simulink model "washout5useful"  (R2018b)
settings: Solver=VariableStepAuto  StartTime=0.0  StopTime=20  RelTol=1e-3
undefined symbols (not defined in the file or in its folder): sigbuilder_block
libraries: fuzblock x2
settings Model: Creator=15705  LastModifiedBy=15705

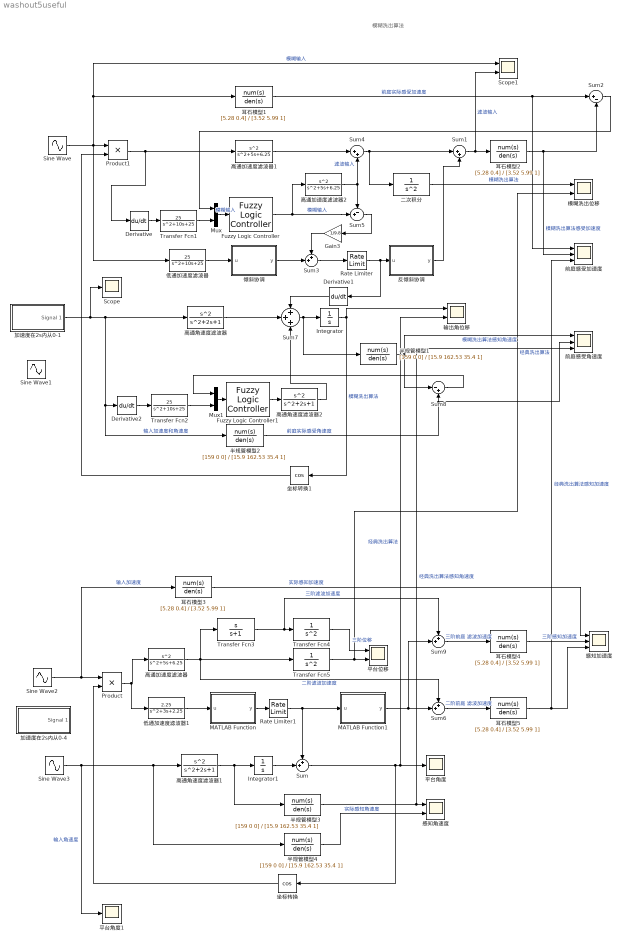
== system washout5useful ==
  note: 模糊洗出算法
  Derivative : Derivative
  Derivative1 : Derivative
  Derivative2 : Derivative
  Fuzzy Logic Controller : fuzblock/Fuzzy Logic  Controller  FIS=InputFuzzy  OutputSampleNumber=101  DataType=double  FuzzifiedInputs=off  RuleFiringStrengths=off  RuleOutputs=off  AggregatedOutputs=off  SimulateUsing=Interpreted execution  OutOfRangeInputValueMessage=warning  NoRuleFiredMessage=warning  EmptyOutputFuzzySetMessage=warning
  Fuzzy Logic Controller1 : fuzblock/Fuzzy Logic  Controller  FIS=Input_ang  OutputSampleNumber=101  DataType=double  FuzzifiedInputs=off  RuleFiringStrengths=off  RuleOutputs=off  AggregatedOutputs=off  SimulateUsing=Interpreted execution  OutOfRangeInputValueMessage=warning  NoRuleFiredMessage=warning  EmptyOutputFuzzySetMessage=warning
  Gain3 : Gain  Gain=1/9.8
  Integrator : Integrator
  Integrator1 : Integrator
  MATLAB Function : MATLAB Function  TreatAsAtomicUnit=on
  MATLAB Function1 : MATLAB Function  TreatAsAtomicUnit=on
  Mux : Mux  Inputs=2
  Mux1 : Mux  Inputs=2
  Product : Product
  Product1 : Product
  Rate Limiter : RateLimiter  RisingSlewLimit=0.0628  FallingSlewLimit=-0.0628  SampleTimeMode=inherited
  Rate Limiter1 : RateLimiter  RisingSlewLimit=0.0628  FallingSlewLimit=-0.0628  SampleTimeMode=inherited
  Scope : Scope
  Scope1 : Scope  NumInputPorts=2
  Sine Wave{,1..3} (4 alike) : Sin  SampleTime=0
  Sum{,3,6,9} (4 alike) : Sum  Inputs=++|
  Sum1 : Sum  Inputs=|++
  Sum2 : Sum  Inputs=|+-
  Sum4 : Sum  Inputs=|++
  Sum5 : Sum  Inputs=-+|
  Sum7 : Sum  Inputs=+++
  Sum8 : Sum  Inputs=|-+
  Transfer Fcn1 : TransferFcn  Numerator=[25]  Denominator=[1 10 25]
  Transfer Fcn2 : TransferFcn  Numerator=[25]  Denominator=[1 10 25]
  Transfer Fcn3 : TransferFcn  Numerator=[1 0]  Denominator=[1 1]
  Transfer Fcn4 : TransferFcn  Denominator=[1 0 0]
  Transfer Fcn5 : TransferFcn  Denominator=[1 0 0]
  二次积分 : TransferFcn  Denominator=[1 0 0]
  低通加速度滤波器 : TransferFcn  Numerator=[25]  Denominator=[1 10 25]
  低通加速度滤波器1 : TransferFcn  Numerator=[2.25]  Denominator=[1 3 2.25]
  倾斜协调 : MATLAB Function  TreatAsAtomicUnit=on
  前庭感受加速度 : Scope  NumInputPorts=3
  前庭感受角速度 : Scope  NumInputPorts=3
  加速度在2s内从0-1 : Subsystem  Tag=STV Subsys  LoadFcn=sigbuilder_block('load');  StartFcn=sigbuilder_block('start');  StopFcn=sigbuilder_block('stop');  ClipboardFcn=sigbuilder_block('clipboard');  mask(Sigbuilder block){tuvar=[0:10]}
      mask help: Simulink:masks:SigbuilderBlock_MD
      mask init:
      | if ~strcmp(get_param(bdroot(gcbh),'SimulationStatus'),'stopped') tuvar = sigbuilder_block('maskInit'); end
      settings: CopyFcn=sigbuilder_block('copy');  DeleteFcn=sigbuilder_block('delete');  ModelCloseFcn=sigbuilder_block('modelClose');  PreSaveFcn=sigbuilder_block('preSave');  PauseFcn=sigbuilder_block('pause');  ContinueFcn=sigbuilder_block('continue');  NameChangeFcn=sigbuilder_block('namechange');  OpenFcn=sigbuilder_block('open',[199.875 127.5 550.5 364.5 ]);  CloseFcn=sigbuilder_block('close');
      mask Display: plot(0, 0, 100, 100,[2, 2, 32, 32, 2], [68, 8, 8, 68, 68],[32, 2], [38, 38], [32, 19, 2],[53, 60, 44], [32, 17, 17, 2],[16, 16, 31, 31]);txt = getActiveGroup(gcbh);text(2, 100, txt,'verticalAlignment', 'top');
  加速度在2s内从0-4 : Subsystem  Tag=STV Subsys  LoadFcn=sigbuilder_block('load');  StartFcn=sigbuilder_block('start');  StopFcn=sigbuilder_block('stop');  ClipboardFcn=sigbuilder_block('clipboard');  mask(Sigbuilder block){tuvar=[0:10]}
      mask help: Simulink:masks:SigbuilderBlock_MD
      mask init:
      | if ~strcmp(get_param(bdroot(gcbh),'SimulationStatus'),'stopped') tuvar = sigbuilder_block('maskInit'); end
      settings: CopyFcn=sigbuilder_block('copy');  DeleteFcn=sigbuilder_block('delete');  ModelCloseFcn=sigbuilder_block('modelClose');  PreSaveFcn=sigbuilder_block('preSave');  PauseFcn=sigbuilder_block('pause');  ContinueFcn=sigbuilder_block('continue');  NameChangeFcn=sigbuilder_block('namechange');  OpenFcn=sigbuilder_block('open',[199.875 127.5 550.5 364.5 ]);  CloseFcn=sigbuilder_block('close');
      mask Display: plot(0, 0, 100, 100,[2, 2, 32, 32, 2], [68, 8, 8, 68, 68],[32, 2], [38, 38], [32, 19, 2],[53, 60, 44], [32, 17, 17, 2],[16, 16, 31, 31]);txt = getActiveGroup(gcbh);text(2, 100, txt,'verticalAlignment', 'top');
  半规管模型{1..4} (4 alike) : TransferFcn  Numerator=[159 0 0]  Denominator=[15.9 162.53 35.4 1]
  反倾斜协调 : MATLAB Function  TreatAsAtomicUnit=on
  坐标转换 : Trigonometry  Operator=cos
  坐标转换1 : Trigonometry  Operator=cos
  平台位移 : Scope  NumInputPorts=2
  平台角度 : Scope
  平台角度1 : Scope
  感知加速度 : Scope  NumInputPorts=3
  感知角速度 : Scope  NumInputPorts=2
  模糊洗出位移 : Scope  NumInputPorts=2
  耳石模型{1..5} (5 alike) : TransferFcn  Numerator=[5.28 0.4]  Denominator=[3.52 5.99 1]
  "输出角位移 " : Scope  NumInputPorts=2
  高通加速度滤波器 : TransferFcn  Numerator=[1 0 0]  Denominator=[1 5 6.25]
  高通加速度滤波器1 : TransferFcn  Numerator=[1 0 0]  Denominator=[1 5 6.25]
  高通加速度滤波器2 : TransferFcn  Numerator=[1 0 0]  Denominator=[1 5 6.25]
  高通角速度滤波器 : TransferFcn  Numerator=[1 0 0]
  高通角速度滤波器1 : TransferFcn  Numerator=[1 0 0]
  高通角速度滤波器2 : TransferFcn  Numerator=[1 0 0]
  wires:
  Rate Limiter/1 -> Derivative1/1, 反倾斜协调/1(u)
  耳石模型2/1 -> Sum2/2, 前庭感受加速度/2  "模糊洗出算法感受加速度"
  二次积分/1 -> 模糊洗出位移/1  "模糊洗出算法"
  耳石模型1/1 -> Sum2/1, 前庭感受加速度/1  "前庭实际感受加速度"
  加速度在2s内从0-1/1(Signal 1) -> Scope/1, 高通角速度滤波器/1, Derivative2/1, 半规管模型2/1  "输入加速度和角速度"
  Sine Wave/1 -> Product1/1, 耳石模型1/1, Scope1/1, 低通加速度滤波器/1  "模糊输入"
  Integrator/1 -> 坐标转换1/1, "输出角位移 "/1  "模糊洗出算法"
  低通加速度滤波器/1 -> 倾斜协调/1(u)
  Mux/1 -> Fuzzy Logic Controller/1  "模糊输入"
  Fuzzy Logic Controller/1 -> 高通加速度滤波器2/1, Sum5/2  "模糊输入"
  倾斜协调/1(y) -> Sum3/2
  Sum3/1 -> Rate Limiter/1
  Derivative/1 -> Transfer Fcn1/1
  高通加速度滤波器1/1 -> Sum4/1
  Sum4/1 -> Sum1/1, 二次积分/1
  高通加速度滤波器2/1 -> Sum5/1, Sum4/2  "滤波输入"
  Sum5/1 -> Gain3/1
  反倾斜协调/1(y) -> Sum1/2
  Sum1/1 -> 耳石模型2/1, Scope1/2  "滤波输入"
  Gain3/1 -> Sum3/1
  Sum2/1 -> Mux/1
  Transfer Fcn1/1 -> Mux/2
  Sum7/1 -> Integrator/1, 半规管模型1/1
  高通角速度滤波器/1 -> Sum7/2
  Derivative1/1 -> Sum7/1
  半规管模型1/1 -> Sum8/1, 前庭感受角速度/1  "模糊洗出算法感知角速度"
  半规管模型2/1 -> 前庭感受角速度/2, Sum8/2  "前庭实际感受角速度"
  Mux1/1 -> Fuzzy Logic Controller1/1
  Derivative2/1 -> Transfer Fcn2/1
  Sum8/1 -> Mux1/1
  Fuzzy Logic Controller1/1 -> 高通角速度滤波器2/1
  高通角速度滤波器2/1 -> Sum7/3
  Transfer Fcn2/1 -> Mux1/2
  半规管模型4/1 -> 感知角速度/2  "实际感知角速度"
  MATLAB Function/1(y) -> Rate Limiter1/1
  高通角速度滤波器1/1 -> 半规管模型3/1, Integrator1/1
  Sum6/1 -> 耳石模型5/1  "二阶前庭 滤波加速度"
  耳石模型4/1 -> 感知加速度/2  "三阶感知加速度"
  低通加速度滤波器1/1 -> MATLAB Function/1(u)
  坐标转换/1 -> Product/2
  半规管模型3/1 -> 前庭感受角速度/3, 感知角速度/1  "经典洗出算法感知角速度"
  MATLAB Function1/1(y) -> Sum9/2, Sum6/2
  Sine Wave2/1 -> Product/1, 耳石模型3/1  "输入加速度"
  耳石模型5/1 -> 前庭感受加速度/3, 感知加速度/3  "经典洗出算法感知加速度"
  Transfer Fcn5/1 -> 模糊洗出位移/2, 平台位移/2  "经典洗出算法"
  耳石模型3/1 -> 感知加速度/1  "实际感知加速度"
  Sum9/1 -> 耳石模型4/1  "三阶前庭 滤波加速度"
  Transfer Fcn3/1 -> Sum9/1, Transfer Fcn4/1  "三阶滤波加速度"
  Integrator1/1 -> Sum/2
  Sine Wave3/1 -> 平台角度1/1, 半规管模型4/1, 高通角速度滤波器1/1  "输入角速度"
  Rate Limiter1/1 -> MATLAB Function1/1(u), Sum/1
  高通加速度滤波器/1 -> Transfer Fcn3/1, Sum6/1, Transfer Fcn5/1  "二阶滤波加速度"
  Product/1 -> 低通加速度滤波器1/1, 高通加速度滤波器/1
  Transfer Fcn4/1 -> 平台位移/1  "三阶位移"
  Sum/1 -> "输出角位移 "/2, 平台角度/1, 坐标转换/1  "经典洗出算法"
  坐标转换1/1 -> Product1/2
  Product1/1 -> Derivative/1, 高通加速度滤波器1/1

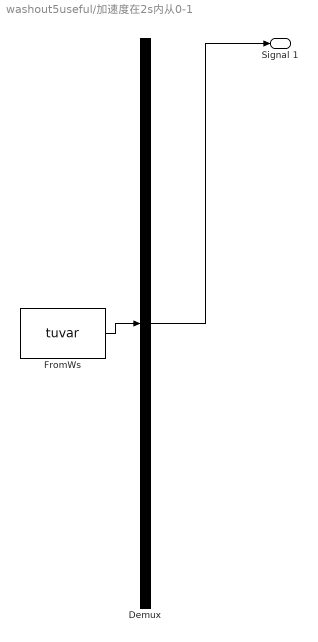
== system washout5useful/加速度在2s内从0-1 ==
  Demux : Demux  Tag=STV Demux  Outputs=1
  FromWs : FromWorkspace  Tag=STV FromWs  VariableName=tuvar  SampleTime=0
      SigBuilderData=|
      | common.afterFinalStr = 'Extrapolate'
      | common.sampleTime = 0
      | dataSet.timeRange = [0 10]
      | dataSet.name = 'Group 1'
      | sbobj.Groups.Name = 'Group 1'
      | sbobj.Groups.Signals.Name = 'Signal 1'
      | sbobj.Groups.Signals.XData = [0 2 3 8 10]
      | sbobj.Groups.Signals.YData = [0 0 1 1 1]
  Signal 1 : Outport  Tag=STV Outport
  wires:
  Demux/1 -> Signal 1/1
  FromWs/1 -> Demux/1

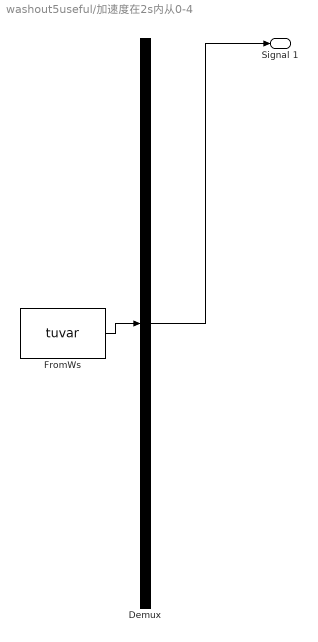
== system washout5useful/加速度在2s内从0-4 ==
  Demux : Demux  Tag=STV Demux  Outputs=1
  FromWs : FromWorkspace  Tag=STV FromWs  VariableName=tuvar  SampleTime=0
      SigBuilderData=|
      | common.afterFinalStr = 'Extrapolate'
      | common.sampleTime = 0
      | dataSet.timeRange = [0 10]
      | dataSet.name = 'Group 1'
      | sbobj.Groups.Name = 'Group 1'
      | sbobj.Groups.Signals.Name = 'Signal 1'
      | sbobj.Groups.Signals.XData = [0 2 3 8 10]
      | sbobj.Groups.Signals.YData = [0 0 1 1 1]
  Signal 1 : Outport  Tag=STV Outport
  wires:
  Demux/1 -> Signal 1/1
  FromWs/1 -> Demux/1

== matlab function washout5useful/反倾斜协调 ==
  data: u input; y output
function y = fcn(u)
y=9.8*sin(u);

== matlab function washout5useful/倾斜协调 ==
  data: u input; y output
function y = fcn(u)
y=asin(u/9.8);

== matlab function washout5useful/MATLAB Function ==
  data: u input; y output
function y = fcn(u)
y=asin(u/9.8);

== matlab function washout5useful/MATLAB Function1 ==
  data: u input; y output
function y = fcn(u)
y=9.8*sin(u);
